simulink model "chap7_1"  (Simulink 3.00)
settings: Solver=ode4  StartTime=0.0  StopTime=2  RelTol=1e-3
values from neighbouring files (symbols this model uses):
  bn = 0.0673    [chap7_1f.m]    (also in chap7_2.m = 0.188)
  bp = 0.067    [chap7_1f.m]    (also in chap7_2.m = 0.188; chap7_5.m = 8)
  Jn = 0.0033    [chap7_1f.m]    (also in chap7_2.m = 0.0075)
  Jp = 0.0030    (= 0.003)    [chap7_1f.m]    (also in chap7_2.m = 0.0075)
  tol = 0.001    [chap7_1f.m]    (also in chap7_2.m = 0.0065)
libraries: simulink_extras x1

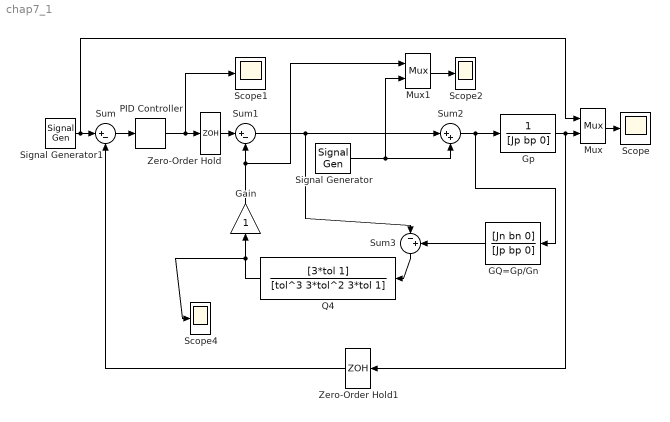
== system chap7_1 ==
  GQ=Gp/Gn : TransferFcn  Orientation=left  Numerator=[Jn bn 0]  Denominator=[Jp bp 0]
  Gain : Gain  Orientation=up  Gain=1  SaturateOnIntegerOverflow=on
  Gp : TransferFcn  Numerator=[1]  Denominator=[Jp bp 0]
  Mux : Mux  Inputs=2
      settings: DisplayOption=none
  Mux1 : Mux  Inputs=2
      settings: DisplayOption=none
  PID Controller : simulink_extras/Additional Linear/PID Controller  P=5  I=0  D=0.5
  Q4 : TransferFcn  Orientation=left  Numerator=[3*tol 1]  Denominator=[tol^3 3*tol^2 3*tol 1]
  Scope{,1..2,4} (4 alike) : Scope
      Scope settings: TimeRange=auto  YMin=-1  YMax=0.5  SaveToWorkspace=off  SaveName=ScopeData  MaxRows=50000
      Scope1 settings: TimeRange=auto  YMin=-5  YMax=5  SaveToWorkspace=off  SaveName=ScopeData  MaxRows=50000
      Scope2 settings: TimeRange=auto  YMin=-5  YMax=5  SaveToWorkspace=off  SaveName=ScopeData  MaxRows=50000
      Scope4 settings: TimeRange=auto  YMin=-5  YMax=5  SaveToWorkspace=off  SaveName=ScopeData  MaxRows=50000
  Signal Generator : SignalGenerator  WaveForm=sine  Amplitude=3  Frequency=5  Units=Hertz
  Signal Generator1 : SignalGenerator  WaveForm=sine  Amplitude=1  Frequency=1  Units=Hertz
  Sum : Sum  Inputs=|+-  SaturateOnIntegerOverflow=on
  Sum1 : Sum  Inputs=|+-  SaturateOnIntegerOverflow=on
  Sum2 : Sum  Inputs=|++  SaturateOnIntegerOverflow=on
  Sum3 : Sum  Orientation=down  Inputs=|-+  SaturateOnIntegerOverflow=on
  Zero-Order Hold : ZeroOrderHold  SampleTime=0.001
  Zero-Order Hold1 : ZeroOrderHold  Orientation=left  SampleTime=0.001
  wires:
  Sum/1 -> PID Controller/1
  Signal Generator1/1 -> Sum/1, Mux/1
  Mux/1 -> Scope/1
  PID Controller/1 -> Scope1/1, Zero-Order Hold/1
  Sum1/1 -> Sum2/1, Sum3/1
  Gp/1 -> Mux/2, Zero-Order Hold1/1
  Sum2/1 -> Gp/1, GQ=Gp/Gn/1
  Mux1/1 -> Scope2/1
  Signal Generator/1 -> Sum2/2, Mux1/2
  Gain/1 -> Sum1/2, Mux1/1
  Zero-Order Hold/1 -> Sum1/1
  Zero-Order Hold1/1 -> Sum/2
  Sum3/1 -> Q4/1
  Q4/1 -> Gain/1, Scope4/1
  GQ=Gp/Gn/1 -> Sum3/2
